simulink library "asbCubeSatFSWLib"  (R2023b)
settings: Solver=VariableStepAuto  StartTime=0.0  StopTime=10.0  RelTol=1e-3
settings Model: Creator=The MathWorks, Inc.  LastModifiedBy=bobow
settings SolverCC: AlgebraicLoopSolver=TrustRegion  MaxZcPerStep=1
settings DebuggingCC: UnconnectedInputMsg=warning  UnconnectedOutputMsg=warning  UnconnectedLineMsg=warning
settings ModelReferenceCC: EnableRefExpFcnMdlSchedulingChecks=on

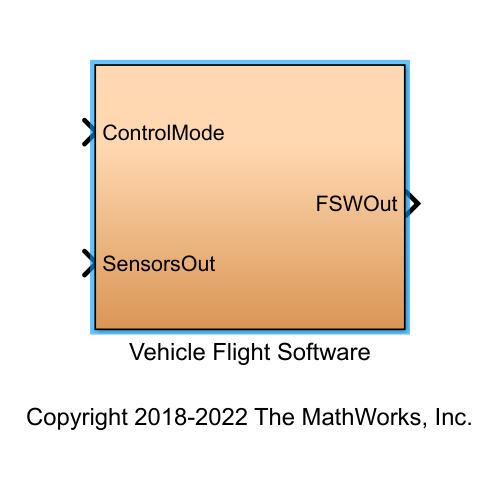
[thumbnail: Simulink's stored preview of the top-level diagram]
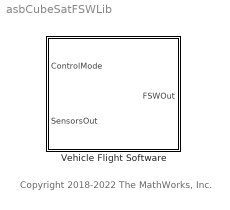
== system asbCubeSatFSWLib ==
  note: Copyright 2018-2022 The MathWorks, Inc.
  Vehicle Flight Software : Subsystem

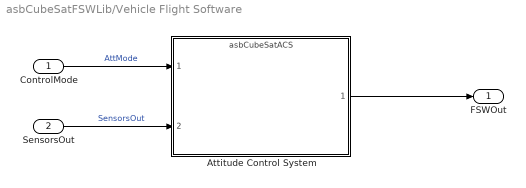
== system asbCubeSatFSWLib/Vehicle Flight Software ==
  ControlMode : Inport
  SensorsOut : Inport  Port=2
  Attitude Control System : ModelReference  ModelNameDialog=asbCubeSatACS.slx  SimulationMode=Normal  ModelReferenceVersion=9.4
  FSWOut : Outport  VectorParamsAs1DForOutWhenUnconnected=off
  wires:
  Attitude Control System/1 -> FSWOut/1
  ControlMode/1 -> Attitude Control System/1  "AttMode"
  SensorsOut/1 -> Attitude Control System/2  "SensorsOut"
